simulink model "FeedforwardBackward_model"  (R2017a)
settings: Solver=VariableStepAuto  StartTime=0.0  StopTime=duur  RelTol=1e-9  EnableMultiTasking=on
values from neighbouring files (symbols this model uses):
  denom_ff = [1 1]    [FeedforwardBackward.m]
  denom_measurement = [3 3]    [FeedforwardBackward.m]
  denom_system = [7 1]    [FeedforwardBackward.m]
  K_c = 1    [FeedforwardBackward.m]
  num_ff = [1]    [FeedforwardBackward.m]
  num_measurement = [-6 -1]    [FeedforwardBackward.m]
  num_system = [3.5]    [FeedforwardBackward.m]
settings Model: Creator=wrquaghe  LastModifiedBy=geert
settings DataIOCC: LimitDataPoints=on
settings OptimizationCC: LifeSpan=inf
settings DebuggingCC: AllowSymbolicDim=off  SFUnexpectedBacktrackingDiag=warning  SFNoUnconditionalDefaultTransitionDiag=warning  SFExecutionAtInitializationDiag=none
settings ModelReferenceCC: PropagateSignalLabelsOutOfModel=off
settings GRTTargetCC: TargetLangStandard=C89/C90 (ANSI)
settings ConfigComp: CovMetricSettings=dw  CovHtmlReporting=on  CovSaveCumulativeToWorkspaceVar=on  CovSaveSingleToWorkspaceVar=on  CovExternalEMLEnable=off

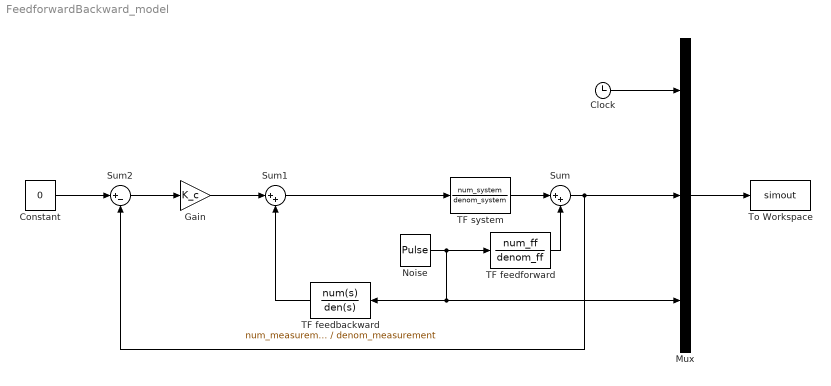
== system FeedforwardBackward_model ==
  Clock : Clock
  Constant : Constant  Value=0
  Gain : Gain  Gain=K_c
  Mux : Mux  Inputs=3
  Noise : DiscretePulseGenerator  Period=10  PulseWidth=5
  Sum : Sum  Inputs=|++
  Sum1 : Sum  Inputs=|++
  Sum2 : Sum  Inputs=|+-
  TF feedbackward : TransferFcn  Numerator=num_measurement  Denominator=denom_measurement
  TF feedforward : TransferFcn  Numerator=num_ff  Denominator=denom_ff
  TF system : TransferFcn  Numerator=num_system  Denominator=denom_system
  To Workspace : ToWorkspace  VariableName=simout  SampleTime=-1
  wires:
  TF system/1 -> Sum/1
  TF feedforward/1 -> Sum/2
  Noise/1 -> Mux/3, TF feedbackward/1, TF feedforward/1
  Clock/1 -> Mux/1
  Mux/1 -> To Workspace/1
  Sum/1 -> Sum2/2, Mux/2
  Gain/1 -> Sum1/1
  Sum2/1 -> Gain/1
  Constant/1 -> Sum2/1
  TF feedbackward/1 -> Sum1/2
  Sum1/1 -> TF system/1
